simulink model "Rsim1"  (R2017a)
settings: Solver=VariableStepAuto  StartTime=0.0  StopTime=10  RelTol=1e-3
values from neighbouring files (symbols this model uses):
  brx = 5    [models.m]
  by = 5    [models.m]
  K = place(A,B,sPoles)    [finalCode.m]
  ki = 36    [models.m]
  kp = 6    [models.m]
  x20 = 0    [finalCode.m]
  yref = 0.12626    [finalCode.m]
settings Model: Creator=rjv  LastModifiedBy=noah
settings OptimizationCC: LifeSpan=inf
settings DebuggingCC: SFExecutionAtInitializationDiag=none
settings SFSimCC: SimUseLocalCustomCode=on
settings RTWCC: RTWUseLocalCustomCode=on

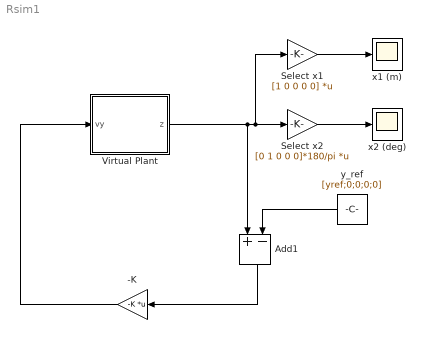
== system Rsim1 ==
  -K : Gain  Gain=-K  Multiplication=Matrix(K*u)
  Add1 : Sum  Inputs=+-
  Select x1 : Gain  Gain=[1 0 0 0 0]  Multiplication=Matrix(K*u)
  Select x2 : Gain  Gain=[0 1 0 0 0]*180/pi  Multiplication=Matrix(K*u)
  Virtual Plant : Subsystem
  x1 (m) : Scope
  x2 (deg) : Scope
  y_ref : Constant  Value=[yref;0;0;0;0]
  wires:
  Select x2/1 -> x2 (deg)/1
  Select x1/1 -> x1 (m)/1
  Virtual Plant/1(z) -> Select x2/1, Select x1/1, Add1/1
  -K/1 -> Virtual Plant/1(vy)
  Add1/1 -> -K/1
  y_ref/1 -> Add1/2

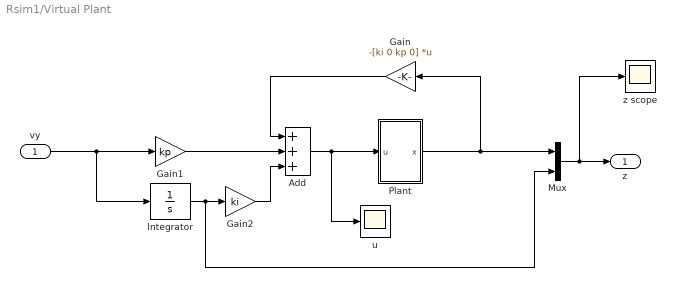
== system Rsim1/Virtual Plant ==
  vy : Inport
  Add : Sum  Inputs=+++
  Gain : Gain  Gain=-[ki 0 kp 0]  Multiplication=Matrix(K*u)
  Gain1 : Gain  Gain=kp
  Gain2 : Gain  Gain=ki
  Mux : Mux  Inputs=2
  Plant : Subsystem
  lntegrator : TransferFcn  Numerator=1  Denominator=[1 0]
  u : Scope
  z scope : Scope
  z : Outport
  wires:
  Gain2/1 -> Add/3
  Gain1/1 -> Add/2
  Plant/1(x) -> Mux/1, Gain/1
  Gain/1 -> Add/1
  Add/1 -> Plant/1(u), u/1
  lntegrator/1 -> Mux/2, Gain2/1
  Mux/1 -> z scope/1, z/1
  vy/1 -> lntegrator/1, Gain1/1

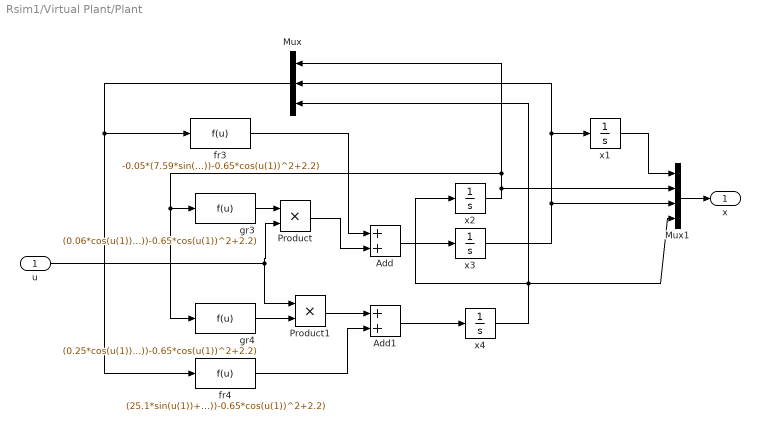
== system Rsim1/Virtual Plant/Plant ==
  u : Inport
  Add : Sum
  Add1 : Sum
  Mux : Mux  Inputs=3
  Mux1 : Mux
  Product : Product
  Product1 : Product
  fr3 : Fcn  Expr=-0.05*(7.59*sin(u(1))-65.5*sin(2*u(1))+11.5*u(3)^2*sin(u(1))+0.45*by*u(2)-0.03*brx*u(3)+0.52*brx*u(3)*cos(u(1)))/(0.075*cos(u(1))-0.65*cos(u(1))^2+2.2)
  fr4 : Fcn  Expr=(25.1*sin(u(1))+0.037*u(3)^2*sin(u(1))-0.32*u(3)^2*sin(2*u(1))-(0.1*brx*u(3)-0.0015*by*u(2)+0.025*by*u(2)*cos(u(1))))/(0.075*cos(u(1))-0.65*cos(u(1))^2+2.2)
  gr3 : Fcn  Expr=(0.06*cos(u(1))+0.21)/(0.075*cos(u(1))-0.65*cos(u(1))^2+2.2)
  gr4 : Fcn  Expr=(0.25*cos(u(1))+0.21)/(0.075*cos(u(1))-0.65*cos(u(1))^2+2.2)
  x1 : Integrator
  x2 : Integrator  InitialCondition=x20
  x3 : Integrator
  x4 : Integrator
  x : Outport
  wires:
  x4/1 -> Mux/3, Mux1/4, x2/1
  x3/1 -> Mux1/3, Mux/2, x1/1
  gr3/1 -> Product/1
  x2/1 -> Mux1/2, Mux/1, gr4/1, gr3/1
  gr4/1 -> Product1/2
  u/1 -> Product/2, Product1/1
  Add/1 -> x3/1
  Add1/1 -> x4/1
  Product1/1 -> Add1/1
  fr4/1 -> Add1/2
  Product/1 -> Add/2
  Mux/1 -> fr3/1, fr4/1
  fr3/1 -> Add/1
  Mux1/1 -> x/1
  x1/1 -> Mux1/1
